simulink model "HDLOFDMSeparator"  (R2024a)
settings: Solver=FixedStepDiscrete  StartTime=0.0  StopTime=stopTime  RelTol=1e-3
values from neighbouring files (symbols this model uses):
  payloadBitsPerSubcarrier = binl2dec(batId)    [parameters.m]
  payloadCyclicPrefixLen = binl2dec(cyclicPrefixId) * CONST.N / 32    [parameters.m]
  psduSizeLSB = flip(psduSize)    [testOFDMSeparator.m]
undefined symbols (not defined in the file or in its folder): fPHY
libraries: HDL_ieee_8021513 x5, whdlutilities x3, dspsrcs4 x2
settings Model: DataTypeOverride=Off  SimulationMode=accelerator  Creator=cotti  LastModifiedBy=cotti
settings OptimizationCC: BlockReduction=off  ConditionallyExecuteInputs=off  DefaultParameterBehavior=Inlined  InheritOutputTypeSmallerThanSingle=on
settings DebuggingCC: ArtificialAlgebraicLoopMsg=error  SingleTaskRateTransMsg=error
settings HardwareCC: ProdBitPerPointer=32  ProdBitPerSizeT=32  ProdBitPerPtrDiffT=32  ProdLargestAtomicFloat=None  ProdIntDivRoundTo=Undefined  ProdEndianess=Unspecified  ProdWordSize=32  ProdHWDeviceType=ASIC/FPGA->ASIC/FPGA  TargetBitPerLong=64  TargetBitPerPointer=64  TargetBitPerSizeT=64  TargetBitPerPtrDiffT=64  TargetLongLongMode=on  TargetIntDivRoundTo=Zero  TargetEndianess=LittleEndian  TargetWordSize=64  TargetHWDeviceType=Custom Processor->MATLAB Host Computer  ProdEqTarget=off

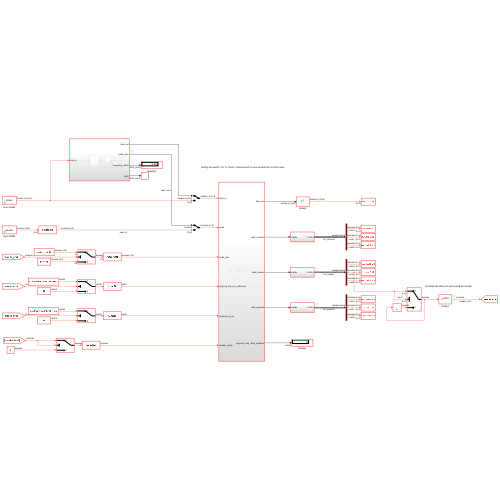
[thumbnail: Simulink's stored preview of the top-level diagram]
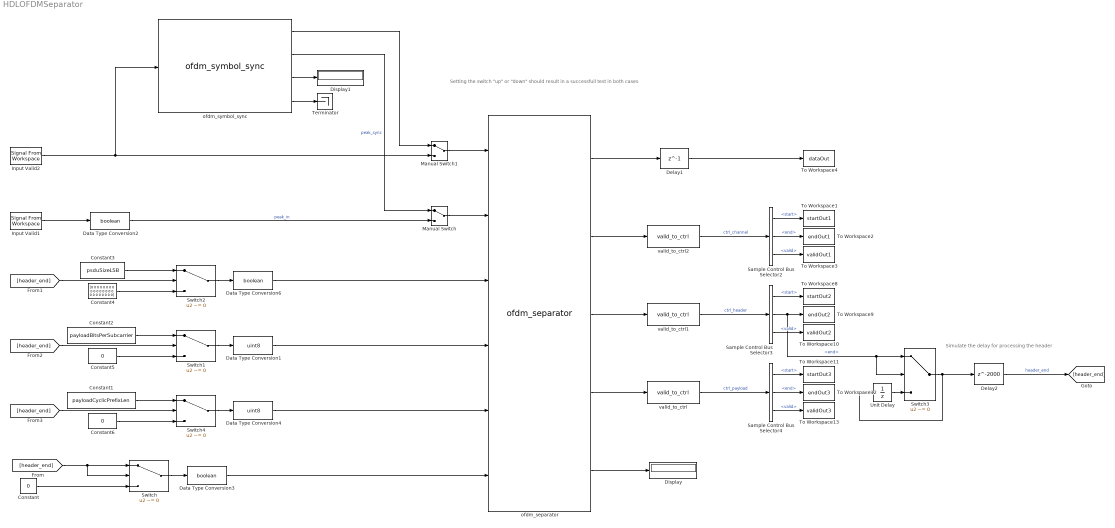
== system HDLOFDMSeparator ==
  note: Setting the switch "up" or "down" should result in a successfull test in both cases
  note: Simulate the delay for processing the header
  Constant : Constant  Value=0  OutDataTypeStr=boolean  SampleTime=1/fPHY
  Constant1 : Constant  Value=payloadCyclicPrefixLen  SampleTime=1/fPHY
  Constant2 : Constant  Value=payloadBitsPerSubcarrier  SampleTime=1/fPHY
  Constant3 : Constant  Value=psduSizeLSB  SampleTime=1/fPHY
  Constant4 : Constant  Value=[0 0 0 0 0 0 0 0 0 0 0 0 0 0 0 0 0 0 0 0 0 0 0 0]  OutDataTypeStr=boolean  SampleTime=1/fPHY
  Constant5 : Constant  Value=0  OutDataTypeStr=uint32  SampleTime=1/fPHY
  Constant6 : Constant  Value=0  OutDataTypeStr=uint32  SampleTime=1/fPHY
  Data Type Conversion1 : DataTypeConversion  OutDataTypeStr=uint8  SaturateOnIntegerOverflow=off  RndMeth=Floor
  Data Type Conversion2 : DataTypeConversion  OutDataTypeStr=boolean  SaturateOnIntegerOverflow=off  RndMeth=Floor
  Data Type Conversion3 : DataTypeConversion  OutDataTypeStr=boolean  SaturateOnIntegerOverflow=off  RndMeth=Floor
  Data Type Conversion4 : DataTypeConversion  OutDataTypeStr=uint8  SaturateOnIntegerOverflow=off  RndMeth=Floor
  Data Type Conversion6 : DataTypeConversion  OutDataTypeStr=boolean  SaturateOnIntegerOverflow=off  RndMeth=Floor
  Delay1 : Delay  DelayLength=1  InitialCondition=0  UseCircularBuffer=on
  Delay2 : Delay  DelayLength=2000  InitialCondition=0  UseCircularBuffer=on
  Display : Display
  Display1 : Display
  Input Valid1 : dspsrcs4/Signal From Workspace  X=peakIn  Ts=1/fPHY  nsamps=1  OutputAfterFinalValue=Setting to zero  ignoreOrWarnInputAndFrameLengths=off  OutputFrames=off
  Input Valid2 : dspsrcs4/Signal From Workspace  X=dataIn  Ts=1/fPHY  nsamps=1  OutputAfterFinalValue=Setting to zero  ignoreOrWarnInputAndFrameLengths=off  OutputFrames=off
  Manual Switch : ManualSwitch
  Manual Switch1 : ManualSwitch
  Sample Control Bus Selector2 : whdlutilities/Sample Control Bus Selector  OutputSignals=start,end,valid
  Sample Control Bus Selector3 : whdlutilities/Sample Control Bus Selector  OutputSignals=start,end,valid
  Sample Control Bus Selector4 : whdlutilities/Sample Control Bus Selector  OutputSignals=start,end,valid
  Switch{,1..4} (5 alike) : Switch  Criteria=u2 ~= 0  SaturateOnIntegerOverflow=off  InputSameDT=off
  Terminator : Terminator
  To Workspace1 : ToWorkspace  VariableName=startOut1  SampleTime=1/fPHY
      settings: Save2DSignal=2-D array (concatenate along first dimension)
  To Workspace10 : ToWorkspace  VariableName=validOut2  SampleTime=1/fPHY
      settings: Save2DSignal=2-D array (concatenate along first dimension)
  To Workspace11 : ToWorkspace  VariableName=startOut3  SampleTime=1/fPHY
      settings: Save2DSignal=2-D array (concatenate along first dimension)
  To Workspace12 : ToWorkspace  VariableName=endOut3  SampleTime=1/fPHY
      settings: Save2DSignal=2-D array (concatenate along first dimension)
  To Workspace13 : ToWorkspace  VariableName=validOut3  SampleTime=1/fPHY
      settings: Save2DSignal=2-D array (concatenate along first dimension)
  To Workspace2 : ToWorkspace  VariableName=endOut1  SampleTime=1/fPHY
      settings: Save2DSignal=2-D array (concatenate along first dimension)
  To Workspace3 : ToWorkspace  VariableName=validOut1  SampleTime=1/fPHY
      settings: Save2DSignal=2-D array (concatenate along first dimension)
  To Workspace4 : ToWorkspace  VariableName=dataOut  SampleTime=1/fPHY
      settings: Save2DSignal=2-D array (concatenate along first dimension)
  To Workspace8 : ToWorkspace  VariableName=startOut2  SampleTime=1/fPHY
      settings: Save2DSignal=2-D array (concatenate along first dimension)
  To Workspace9 : ToWorkspace  VariableName=endOut2  SampleTime=1/fPHY
      settings: Save2DSignal=2-D array (concatenate along first dimension)
  Unit Delay : UnitDelay  SampleTime=-1  HasFrameUpgradeWarning=on
  ofdm_separator : HDL_ieee_8021513/ofdm_separator  SystemSampleTime=-1  VariantActivationTime=update diagram  AllowFlexibleInterface=on  Latency=0  AutoFrameSizeCalculation=off
      settings: SourceProductName=HDL IEEE 8021513
  ofdm_symbol_sync : HDL_ieee_8021513/ofdm_symbol_sync  SystemSampleTime=-1  VariantActivationTime=update diagram  AllowFlexibleInterface=on  Latency=0  AutoFrameSizeCalculation=off
      settings: SourceProductName=HDL IEEE 8021513
  valid_to_ctrl : HDL_ieee_8021513/valid_to_ctrl  SystemSampleTime=-1  VariantActivationTime=update diagram  AllowFlexibleInterface=on  Latency=0  AutoFrameSizeCalculation=off
      settings: SourceProductName=HDL IEEE 8021513
  valid_to_ctrl1 : HDL_ieee_8021513/valid_to_ctrl  SystemSampleTime=-1  VariantActivationTime=update diagram  AllowFlexibleInterface=on  Latency=0  AutoFrameSizeCalculation=off
      settings: SourceProductName=HDL IEEE 8021513
  valid_to_ctrl2 : HDL_ieee_8021513/valid_to_ctrl  SystemSampleTime=-1  VariantActivationTime=update diagram  AllowFlexibleInterface=on  Latency=0  AutoFrameSizeCalculation=off
      settings: SourceProductName=HDL IEEE 8021513
  wires:
  Input Valid1/1 -> Data Type Conversion2/1
  ofdm_separator/4 -> valid_to_ctrl/1
  ofdm_separator/3 -> valid_to_ctrl1/1
  ofdm_separator/2 -> valid_to_ctrl2/1
  ofdm_separator/1 -> Delay1/1
  Delay1/1 -> To Workspace4/1
  Sample Control Bus Selector2/3 -> To Workspace3/1  "<valid>"
  Sample Control Bus Selector2/1 -> To Workspace1/1  "<start>"
  valid_to_ctrl2/1 -> Sample Control Bus Selector2/1  "ctrl_channel"
  Sample Control Bus Selector2/2 -> To Workspace2/1  "<end>"
  Sample Control Bus Selector3/3 -> To Workspace10/1  "<valid>"
  Sample Control Bus Selector3/1 -> To Workspace8/1  "<start>"
  valid_to_ctrl1/1 -> Sample Control Bus Selector3/1  "ctrl_header"
  Sample Control Bus Selector4/3 -> To Workspace13/1  "<valid>"
  Sample Control Bus Selector4/1 -> To Workspace11/1  "<start>"
  Sample Control Bus Selector4/2 -> To Workspace12/1  "<end>"
  valid_to_ctrl/1 -> Sample Control Bus Selector4/1  "ctrl_payload"
  ofdm_separator/5 -> Display/1
  Input Valid2/1 -> ofdm_symbol_sync/1, Manual Switch1/2
  ofdm_symbol_sync/3 -> Display1/1
  ofdm_symbol_sync/4 -> Terminator/1
  ofdm_symbol_sync/1 -> Manual Switch1/1
  Manual Switch1/1 -> ofdm_separator/1
  ofdm_symbol_sync/2 -> Manual Switch/1  "peak_sync"
  Data Type Conversion2/1 -> Manual Switch/2  "peak_in"
  Manual Switch/1 -> ofdm_separator/2
  Unit Delay/1 -> Switch3/3
  Delay2/1 -> [header_end]  "header_end"
  Switch3/1 -> Delay2/1, Unit Delay/1
  Sample Control Bus Selector3/2 -> Switch3/1, Switch3/2, To Workspace9/1  "<end>"
  Constant3/1 -> Switch2/1
  Constant5/1 -> Switch1/3
  Switch1/1 -> Data Type Conversion1/1
  Data Type Conversion3/1 -> ofdm_separator/6
  [header_end] -> Switch2/2
  [header_end] -> Switch/2, Switch/1
  Constant2/1 -> Switch1/1
  Switch2/1 -> Data Type Conversion6/1
  [header_end] -> Switch1/2
  Data Type Conversion1/1 -> ofdm_separator/4
  Constant/1 -> Switch/3
  Constant4/1 -> Switch2/3
  Switch/1 -> Data Type Conversion3/1
  Data Type Conversion6/1 -> ofdm_separator/3
  Switch4/1 -> Data Type Conversion4/1
  Constant6/1 -> Switch4/3
  Data Type Conversion4/1 -> ofdm_separator/5
  Constant1/1 -> Switch4/1
  [header_end] -> Switch4/2
